simulink model "stateFeedback"  (R2025b)
settings: Solver=VariableStepAuto  StartTime=0.0  StopTime=10.0  RelTol=1e-3
settings Model: Creator=g3sha  LastModifiedBy=g3sha

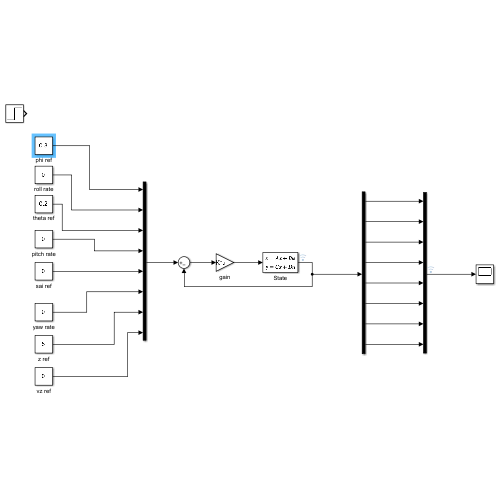
[thumbnail: Simulink's stored preview of the top-level diagram]
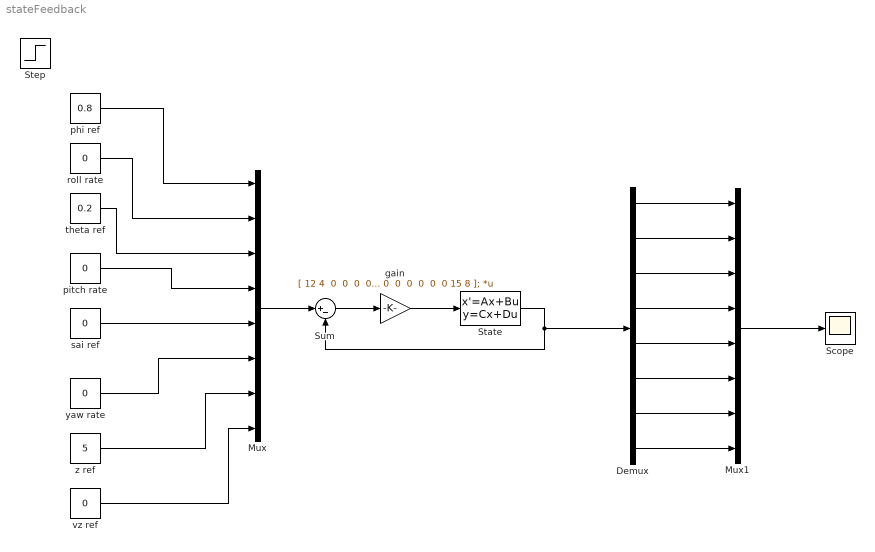
== system stateFeedback ==
  Demux : Demux  Outputs=8
  Mux : Mux  Inputs=8
  Mux1 : Mux  Inputs=8
  Scope : Scope
  State : StateSpace  A=|  B=|  C=eye(8);  D=zeros(8,4);  InitialCondition=0
      A=|
      | [0 1 0 0 0 0 0 0;
      | 0 0 0 0 0 0 0 0;
      | 0 0 0 1 0 0 0 0;
      | 0 0 0 0 0 0 0 0;
      | 0 0 0 0 0 1 0 0;
      | 0 0 0 0 0 0 0 0;
      | 0 0 0 0 0 0 0 1;
      | 0 0 0 0 0 0 0 0];
      B=|
      | [0  0  0 0;
      | 50 0  0 0;
      | 0  0  0 0;
      | 0 50  0 0;
      | 0  0  0 0;
      | 0  0 25 0;
      | 0  0  0 0;
      | 0  0  0 1];
  Step : Step  SampleTime=0
  Sum : Sum  Inputs=|+-
  gain : Gain  Gain=|  Multiplication=Matrix(K*u)
      | [
      | 12 4  0  0  0  0  0  0;
      | 0  0 12 4  0  0  0  0;
      | 0  0  0  0  8  3  0  0;
      | 0  0  0  0  0  0 15 8
      | ];
  phi ref : Constant  Value=0.8
  pitch rate : Constant  Value=0
  roll rate : Constant  Value=0
  sai ref : Constant  Value=0
  theta ref : Constant  Value=0.2
  vz ref : Constant  Value=0
  yaw rate : Constant  Value=0
  z ref : Constant  Value=5
  wires:
  phi ref/1 -> Mux/1
  roll rate/1 -> Mux/2
  theta ref/1 -> Mux/3
  pitch rate/1 -> Mux/4
  sai ref/1 -> Mux/5
  yaw rate/1 -> Mux/6
  z ref/1 -> Mux/7
  vz ref/1 -> Mux/8
  Mux/1 -> Sum/1
  State/1 -> Demux/1, Sum/2
  Sum/1 -> gain/1
  gain/1 -> State/1
  Demux/1 -> Mux1/1
  Demux/2 -> Mux1/2
  Demux/3 -> Mux1/3
  Demux/4 -> Mux1/4
  Demux/5 -> Mux1/5
  Demux/6 -> Mux1/6
  Demux/7 -> Mux1/7
  Demux/8 -> Mux1/8
  Mux1/1 -> Scope/1
